simulink model "HKMASH111_20251011"  (R2024b)
settings: Solver=VariableStepAuto  StartTime=0.0  StopTime=300  RelTol=1e-3
settings Model: Creator=gjp88  LastModifiedBy=gjp88

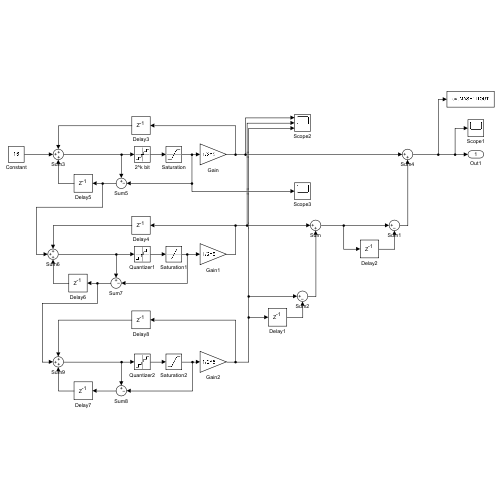
[thumbnail: Simulink's stored preview of the top-level diagram]
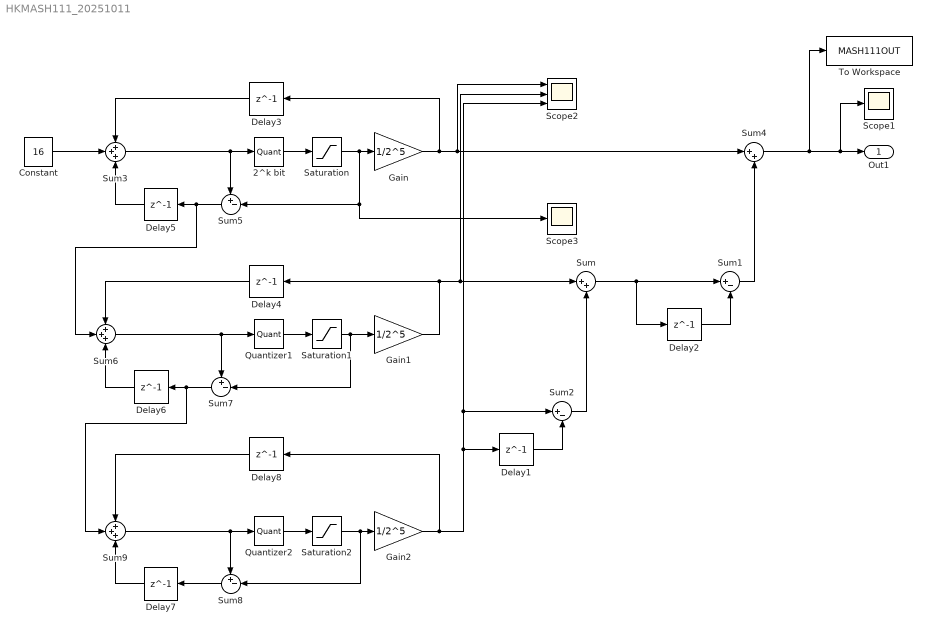
== system HKMASH111_20251011 ==
  2^k bit : Quantizer  QuantizationInterval=2^5
  Constant : Constant  Value=16  SampleTime=0.1
  Delay{1..8} (8 alike) : Delay  DelayLength=1  InitialCondition=0
  Gain : Gain  Gain=1/2^5
  Gain1 : Gain  Gain=1/2^5
  Gain2 : Gain  Gain=1/2^5
  Quantizer1 : Quantizer  QuantizationInterval=2^5
  Quantizer2 : Quantizer  QuantizationInterval=2^5
  Saturation : Saturate  UpperLimit=2^5  LowerLimit=-2^5
  Saturation1 : Saturate  UpperLimit=2^5  LowerLimit=-2^5
  Saturation2 : Saturate  UpperLimit=2^5  LowerLimit=-2^5
  Scope1 : Scope
  Scope2 : Scope  NumInputPorts=3
  Scope3 : Scope
  Sum : Sum  Inputs=|++  SaturateOnIntegerOverflow=on
  Sum1 : Sum  Inputs=|+-
  Sum2 : Sum  Inputs=|+-
  Sum3 : Sum  Inputs=+++
  Sum4 : Sum  Inputs=|++
  Sum5 : Sum  Inputs=+-|
  Sum6 : Sum  Inputs=+++
  Sum7 : Sum  Inputs=+-|
  Sum8 : Sum  Inputs=+-|
  Sum9 : Sum  Inputs=+++
  To Workspace : ToWorkspace  VariableName=MASH111OUT  SampleTime=-1
  Out1 : Outport
  wires:
  Constant/1 -> Sum3/2
  Sum7/1 -> Sum9/2, Delay6/1
  Sum1/1 -> Sum4/2
  Delay1/1 -> Sum2/2
  Sum2/1 -> Sum/2
  Sum/1 -> Sum1/1, Delay2/1
  Delay2/1 -> Sum1/2
  Delay5/1 -> Sum3/3
  Sum3/1 -> 2^k bit/1, Sum5/1
  Sum5/1 -> Sum6/2, Delay5/1
  Sum6/1 -> Quantizer1/1, Sum7/1
  Delay6/1 -> Sum6/3
  Sum9/1 -> Quantizer2/1, Sum8/1
  Sum8/1 -> Delay7/1
  Delay7/1 -> Sum9/3
  Sum4/1 -> To Workspace/1, Out1/1, Scope1/1
  2^k bit/1 -> Saturation/1
  Quantizer2/1 -> Saturation2/1
  Quantizer1/1 -> Saturation1/1
  Saturation/1 -> Gain/1, Scope3/1, Sum5/2
  Saturation1/1 -> Gain1/1, Sum7/2
  Saturation2/1 -> Gain2/1, Sum8/2
  Delay3/1 -> Sum3/1
  Gain/1 -> Delay3/1, Scope2/1, Sum4/1
  Gain1/1 -> Delay4/1, Scope2/2, Sum/1
  Delay4/1 -> Sum6/1
  Delay8/1 -> Sum9/1
  Gain2/1 -> Delay8/1, Scope2/3, Sum2/1, Delay1/1
